simulink model "Acceleration_ANTTAY001"  (R2020a)
settings: Solver=ode4  StartTime=0.0  StopTime=45  FixedStep=0.2  RelTol=1e-3
model workspace (MAT data in the model file):
  alpha_gain = Simulink.Parameter
  alpha_gain.DataType = 'auto'
  alpha_gain.Dimensions = [0 0]
undefined symbols (not defined in the file or in its folder): K
settings Model: Creator=KNMALE002  LastModifiedBy=Tayla
settings DataIOCC: SaveOutput=off  SignalLogging=off  DSMLogging=off  ReturnWorkspaceOutputs=off  TimeSaveName=simulation_time
settings DebuggingCC: ArithmeticOperatorsInVariantConditions=warning
settings SFSimCC: CustomCodeUndefinedFunction=UseInterfaceOnly

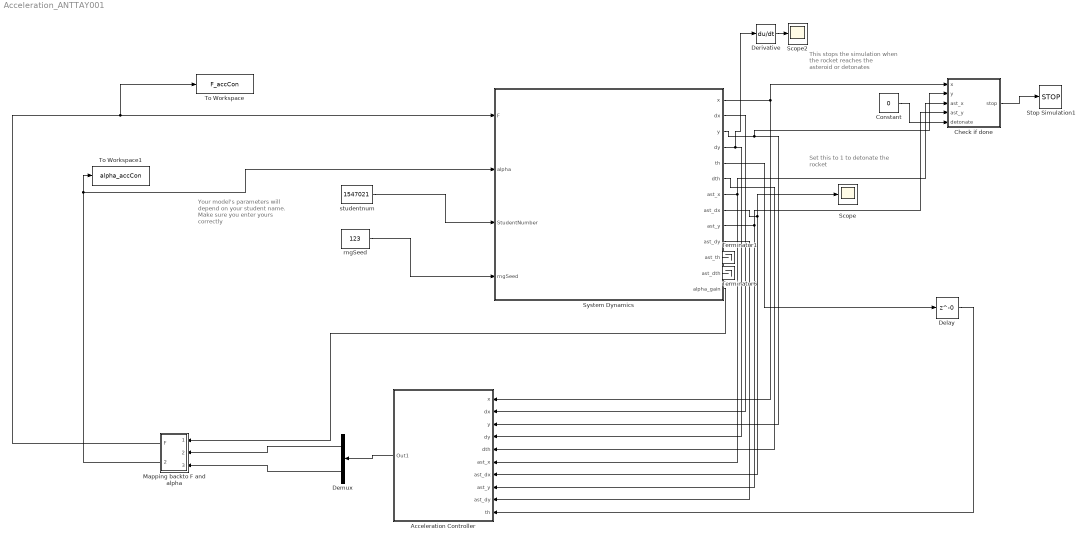
== system Acceleration_ANTTAY001 ==
  note: Your model's parameters will depend on your student name. Make sure you enter yours correctly
  note: This stops the simulation when the rocket reaches the asteroid or detonates
  note: Set this to 1 to detonate the rocket
  Acceleration Controller : Subsystem
  Check if done : MATLAB Function  TreatAsAtomicUnit=on
  Constant : Constant  Value=0
  Delay : Delay  DelayLength=0  InitialCondition=-pi/8
  Demux : Demux  Outputs=2
  Derivative : Derivative
  Mapping backto F and alpha : Subsystem
  Scope : Scope
  Scope2 : Scope
  Stop Simulation1 : Stop
  System Dynamics : Subsystem  TreatAsAtomicUnit=on  mask{Value=1}
      mask prompts: Value "Enter mode (1, 2 or 3)"
      mask TypeOptions Value: ScenarioVar/Value
      mask Display: image('lander.jpg');
  Terminator1 : Terminator
  Terminator6 : Terminator
  To Workspace : ToWorkspace  VariableName=F_accCon  SaveFormat=Timeseries  SampleTime=-1
  To Workspace1 : ToWorkspace  VariableName=alpha_accCon  SaveFormat=Timeseries  SampleTime=-1
  rngSeed : Constant  Value=123
  studentnum : Constant  Value=1547021
  wires:
  studentnum/1 -> System Dynamics/3(StudentNumber)
  System Dynamics/1(x) -> Check if done/1(x), Acceleration Controller/1(x)
  rngSeed/1 -> System Dynamics/4(rngSeed)
  System Dynamics/3(y) -> Acceleration Controller/3(y), Check if done/2(y)
  System Dynamics/9(ast_y) -> Check if done/4(ast_y), Acceleration Controller/8(ast_y)
  System Dynamics/8(ast_dx) -> Acceleration Controller/7(ast_dx), Scope/1
  Check if done/1(stop) -> Stop Simulation1/1
  Constant/1 -> Check if done/5(detonate)
  System Dynamics/4(dy) -> Derivative/1, Acceleration Controller/4(dy)
  Derivative/1 -> Scope2/1
  System Dynamics/7(ast_x) -> Acceleration Controller/6(ast_x), Check if done/3(ast_x)
  System Dynamics/11(ast_th) -> Terminator1/1
  System Dynamics/5(th) -> Delay/1
  System Dynamics/12(ast_dth) -> Terminator6/1
  System Dynamics/2(dx) -> Acceleration Controller/2(dx)
  System Dynamics/6(dth) -> Acceleration Controller/5(dth)
  System Dynamics/10(ast_dy) -> Acceleration Controller/9(ast_dy)
  Delay/1 -> Acceleration Controller/10(th)
  Acceleration Controller/1(Out1) -> Demux/1
  Mapping backto F and alpha/2(alpha) -> To Workspace1/1, System Dynamics/2(alpha)
  System Dynamics/13(alpha_gain) -> Mapping backto F and alpha/1(In1)
  Demux/1 -> Mapping backto F and alpha/2(In2)
  Demux/2 -> Mapping backto F and alpha/3(In3)
  Mapping backto F and alpha/1(F) -> System Dynamics/1(F), To Workspace/1

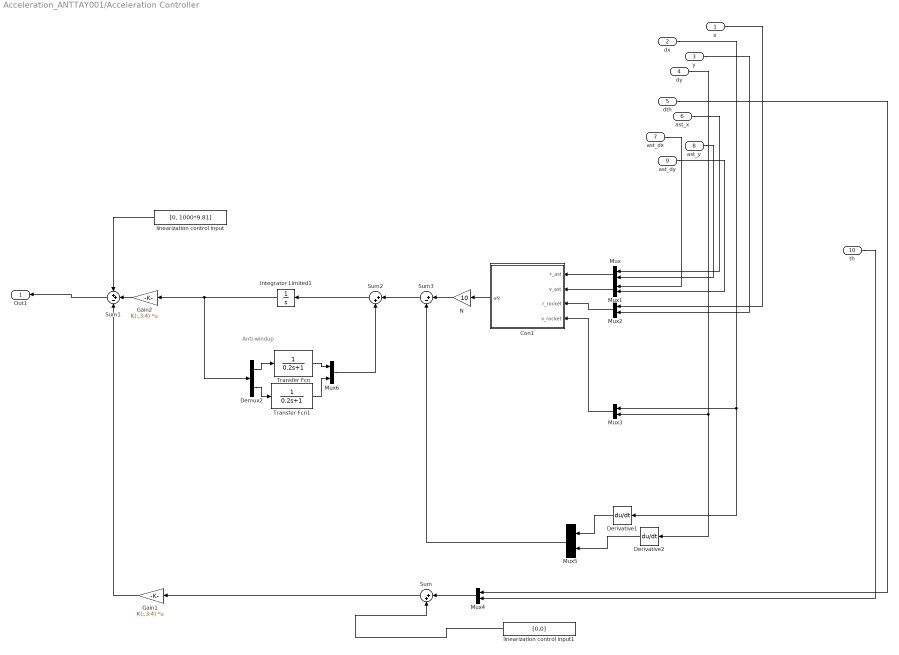
== system Acceleration_ANTTAY001/Acceleration Controller ==
  note: Anti-windup
  x : Inport
  dx : Inport  Port=2
  y : Inport  Port=3
  dy : Inport  Port=4
  dth : Inport  Port=5
  ast_x : Inport  Port=6
  ast_dx : Inport  Port=7
  ast_y : Inport  Port=8
  ast_dy : Inport  Port=9
  th : Inport  Port=10
  Con1 : MATLAB Function  TreatAsAtomicUnit=on
  Demux2 : Demux  Outputs=2
  Derivative1 : Derivative
  Derivative2 : Derivative
  Gain1 : Gain  Gain=K(:,3:4)  Multiplication=Matrix(K*u)
  Gain2 : Gain  Gain=K(:,3:4)  Multiplication=Matrix(K*u)
  Integrator Limited1 : Integrator  LimitOutput=on  UpperSaturationLimit=[8, 965]  LowerSaturationLimit=0
  Mux{,1..6} (7 alike) : Mux  Inputs=2
  N : Gain  Gain=10
  Sum : Sum  Inputs=|++
  Sum1 : Sum  Inputs=++-
  Sum2 : Sum  Inputs=|++
  Sum3 : Sum  Inputs=|+-
  Transfer Fcn : TransferFcn  Denominator=[0.2 1]
  Transfer Fcn1 : TransferFcn  Denominator=[0.2 1]
  linearization control input : Constant  Value=[0, 1000*9.81]
  linearization control input1 : Constant  Value=[0,0]
  Out1 : Outport
  wires:
  Mux5/1 -> Sum3/2
  Mux3/1 -> Con1/4(v_rocket)
  N/1 -> Sum3/1
  Mux/1 -> Con1/1(r_ast)
  Gain1/1 -> Sum1/3
  Mux1/1 -> Con1/2(v_ast)
  dy/1 -> Derivative2/1, Mux3/2
  Mux2/1 -> Con1/3(r_rocket)
  dx/1 -> Derivative1/1, Mux3/1
  dth/1 -> Mux4/1
  Gain2/1 -> Sum1/2
  ast_dx/1 -> Mux1/1
  Mux4/1 -> Sum/1
  Con1/1(aN) -> N/1
  y/1 -> Mux2/2
  Sum3/1 -> Sum2/1
  Derivative2/1 -> Mux5/2
  Derivative1/1 -> Mux5/1
  ast_dy/1 -> Mux1/2
  Sum2/1 -> Integrator Limited1/1
  linearization control input/1 -> Sum1/1
  x/1 -> Mux2/1
  linearization control input1/1 -> Sum/2
  Sum/1 -> Gain1/1
  ast_y/1 -> Mux/2
  ast_x/1 -> Mux/1
  Sum1/1 -> Out1/1
  th/1 -> Mux4/2
  Mux6/1 -> Sum2/2
  Transfer Fcn/1 -> Mux6/1
  Demux2/2 -> Transfer Fcn1/1
  Demux2/1 -> Transfer Fcn/1
  Integrator Limited1/1 -> Demux2/1, Gain2/1
  Transfer Fcn1/1 -> Mux6/2

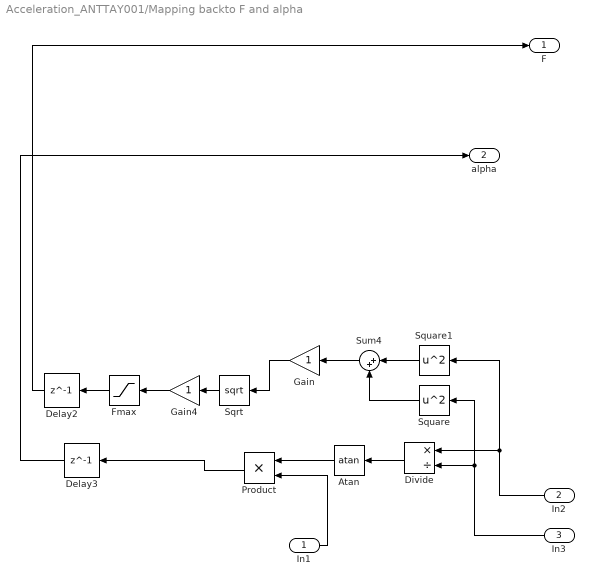
== system Acceleration_ANTTAY001/Mapping backto F and alpha ==
  In1 : Inport
  In2 : Inport  Port=2
  In3 : Inport  Port=3
  Atan : Trigonometry  Operator=atan
  Delay2 : Delay  DelayLength=1  InitialCondition=10000000000
  Delay3 : Delay  DelayLength=1
  Divide : Product  Inputs=*/
  Fmax : Saturate  UpperLimit=39250  LowerLimit=0
  Gain : Gain
  Gain4 : Gain
  Product : Product
  Sqrt : Sqrt  SaturateOnIntegerOverflow=on
  Square : Math  Operator=square  SignedPower=on  SaturateOnIntegerOverflow=on
  Square1 : Math  Operator=square  SignedPower=on  SaturateOnIntegerOverflow=on
  Sum4 : Sum  Inputs=|++
  F : Outport
  alpha : Outport  Port=2
  wires:
  Fmax/1 -> Delay2/1
  Sqrt/1 -> Gain4/1
  Divide/1 -> Atan/1
  In2/1 -> Divide/1, Square1/1
  Square1/1 -> Sum4/1
  Atan/1 -> Product/1
  Gain/1 -> Sqrt/1
  Sum4/1 -> Gain/1
  In3/1 -> Divide/2, Square/1
  Square/1 -> Sum4/2
  Gain4/1 -> Fmax/1
  Delay2/1 -> F/1
  Delay3/1 -> alpha/1
  Product/1 -> Delay3/1
  In1/1 -> Product/2

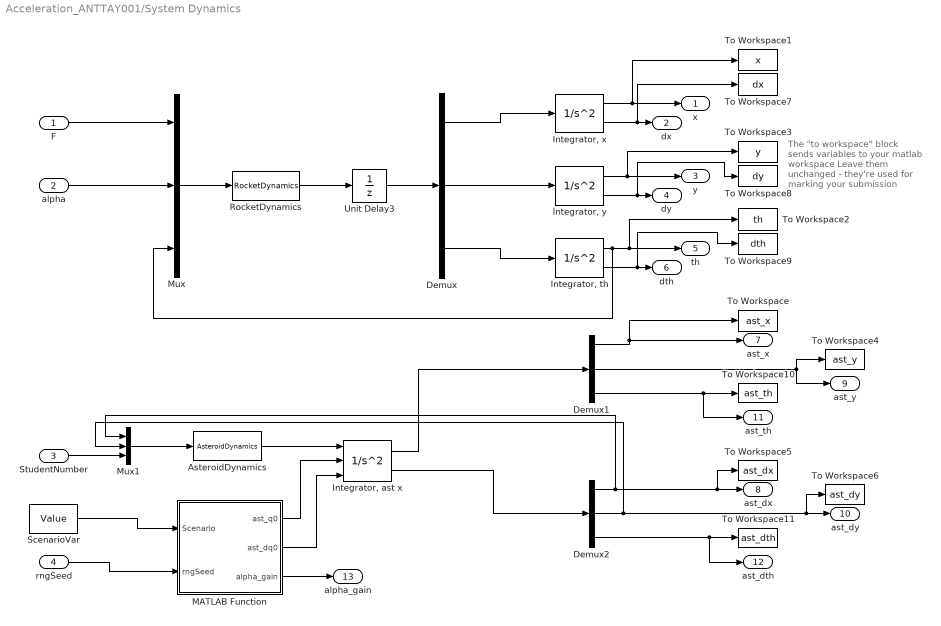
== system Acceleration_ANTTAY001/System Dynamics ==
  note: The "to workspace" block sends variables to your matlab workspace
      |
      | Leave them unchanged - they're used for marking your submission
  F : Inport
  alpha : Inport  Port=2
  StudentNumber : Inport  Port=3
  rngSeed : Inport  Port=4
  AsteroidDynamics : MATLABFcn  MATLABFcn=AsteroidDynamics  OutputDimensions=3
  Demux : Demux  Outputs=3
  Demux1 : Demux  Outputs=3
  Demux2 : Demux  Outputs=3
  "Integrator, th" : SecondOrderIntegrator  ICX=0  ICDXDT=0
  "Integrator, x" : SecondOrderIntegrator  ICX=0
  "Integrator, y" : SecondOrderIntegrator  ICX=0
  "Integrator, ast x" : SecondOrderIntegrator  ICSourceX=external  ICX=x0  ICSourceDXDT=external
  MATLAB Function : MATLAB Function  TreatAsAtomicUnit=on
  Mux : Mux  Inputs=3
  Mux1 : Mux  Inputs=3
  RocketDynamics : MATLABFcn  MATLABFcn=RocketDynamics  Output1D=off
  ScenarioVar : Constant  Value=Value
  To Workspace : ToWorkspace  VariableName=ast_x  SampleTime=-1
  To Workspace1 : ToWorkspace  VariableName=x  SampleTime=-1
  To Workspace10 : ToWorkspace  VariableName=ast_th  SampleTime=-1
  To Workspace11 : ToWorkspace  VariableName=ast_dth  SampleTime=-1
  To Workspace2 : ToWorkspace  VariableName=th  SampleTime=-1
  To Workspace3 : ToWorkspace  VariableName=y  SampleTime=-1
  To Workspace4 : ToWorkspace  VariableName=ast_y  SampleTime=-1
  To Workspace5 : ToWorkspace  VariableName=ast_dx  SampleTime=-1
  To Workspace6 : ToWorkspace  VariableName=ast_dy  SampleTime=-1
  To Workspace7 : ToWorkspace  VariableName=dx  SampleTime=-1
  To Workspace8 : ToWorkspace  VariableName=dy  SampleTime=-1
  To Workspace9 : ToWorkspace  VariableName=dth  SampleTime=-1
  Unit Delay3 : UnitDelay  SampleTime=-1  HasFrameUpgradeWarning=on
  x : Outport  PortDimensions=1  VectorParamsAs1DForOutWhenUnconnected=off
  dx : Outport  Port=2  PortDimensions=1  VectorParamsAs1DForOutWhenUnconnected=off
  y : Outport  Port=3  PortDimensions=1  VectorParamsAs1DForOutWhenUnconnected=off
  dy : Outport  Port=4  PortDimensions=1  VectorParamsAs1DForOutWhenUnconnected=off
  th : Outport  Port=5  PortDimensions=1  VectorParamsAs1DForOutWhenUnconnected=off
  dth : Outport  Port=6  PortDimensions=1  VectorParamsAs1DForOutWhenUnconnected=off
  ast_x : Outport  Port=7  PortDimensions=1  VectorParamsAs1DForOutWhenUnconnected=off
  ast_dx : Outport  Port=8  PortDimensions=1  VectorParamsAs1DForOutWhenUnconnected=off
  ast_y : Outport  Port=9  PortDimensions=1  VectorParamsAs1DForOutWhenUnconnected=off
  ast_dy : Outport  Port=10  PortDimensions=1  VectorParamsAs1DForOutWhenUnconnected=off
  ast_th : Outport  Port=11  PortDimensions=1  VectorParamsAs1DForOutWhenUnconnected=off
  ast_dth : Outport  Port=12  PortDimensions=1  VectorParamsAs1DForOutWhenUnconnected=off
  alpha_gain : Outport  Port=13
  wires:
  "Integrator, th"/1 -> th/1, To Workspace2/1, Mux/3
  Demux/1 -> "Integrator, x"/1
  Demux/2 -> "Integrator, y"/1
  Demux/3 -> "Integrator, th"/1
  "Integrator, x"/1 -> x/1, To Workspace1/1
  "Integrator, x"/2 -> To Workspace7/1, dx/1
  "Integrator, y"/2 -> To Workspace8/1, dy/1
  "Integrator, th"/2 -> To Workspace9/1, dth/1
  Mux/1 -> RocketDynamics/1
  RocketDynamics/1 -> Unit Delay3/1
  rngSeed/1 -> MATLAB Function/2(rngSeed)
  ScenarioVar/1 -> MATLAB Function/1(Scenario)
  F/1 -> Mux/1
  alpha/1 -> Mux/2
  Demux1/2 -> To Workspace4/1, ast_y/1
  Demux1/3 -> To Workspace10/1, ast_th/1
  Demux2/3 -> ast_dth/1, To Workspace11/1
  Mux1/1 -> AsteroidDynamics/1
  AsteroidDynamics/1 -> "Integrator, ast x"/1
  "Integrator, ast x"/1 -> Demux1/1
  "Integrator, ast x"/2 -> Demux2/1
  Demux1/1 -> To Workspace/1, ast_x/1
  Demux2/1 -> Mux1/1, To Workspace5/1, ast_dx/1
  Demux2/2 -> Mux1/2, To Workspace6/1, ast_dy/1
  MATLAB Function/1(ast_q0) -> "Integrator, ast x"/2
  MATLAB Function/2(ast_dq0) -> "Integrator, ast x"/3
  StudentNumber/1 -> Mux1/3
  Unit Delay3/1 -> Demux/1
  "Integrator, y"/1 -> y/1, To Workspace3/1
  MATLAB Function/3(alpha_gain) -> alpha_gain/1

== matlab function Acceleration_ANTTAY001/System Dynamics/MATLAB Function ==
  data: ast_q0 output; ast_dq0 output; Scenario input; rngSeed input; alpha_gain output
function [ast_q0, ast_dq0,alpha_gain] = fcn(Scenario, rngSeed)
rng(rngSeed);
alpha_gain = 1;

if (Scenario == 1)
    x0 = -3000;
    y0 =  5000;
    th0 =   0;
    dx0 = 182;
    dy0 = 0;
    dth0 = 0;
    alpha_gain = 1/10;
    
elseif (Scenario == 2)
    x0 = -2000 + rand_within_plus_minus(100);
    y0 = 4000 + rand_within_plus_minus(100); 
    th0 = 0;
    dx0 = 170;
    dy0 = 0;
    dth0 = 0.1;
    alpha_gain = 1;

elseif (Scenario == 3)
    x0 = -2500;
    y0 = 3000;
    th0 = 0;
    dx0 = 160;
    dy0 = 100;
    dth0 = deg2rad(rand_within_plus_minus(20)); % rad/sec
    theta_in = -pi/8;
    alpha_gain =1;
else
    error('You entered an invalid mode -- make sure Scenario = 1, 2 or 3')
end

alpha_gain = alpha_gain;
ast_q0  = [ x0;  y0;  th0];
ast_dq0 = [dx0; dy0; dth0];

end

% calling rand_within_plus_minus(100) returns a number between -100 and 100
function n = rand_within_plus_minus(interval)
    n = (rand - 0.5) * 2 * interval;
end

== matlab function Acceleration_ANTTAY001/Acceleration Controller/Con1 ==
  data: r_ast input; aN output size=2; v_ast input; r_rocket input; v_rocket input
function aN = pNav(r_ast, v_ast, r_rocket, v_rocket)
% https://en.wikipedia.org/wiki/Proportional_navigation
% this produces an acceleration which the controller should track
R = r_ast - r_rocket;
Rtemp = [R; 0];
Vr = v_ast - v_rocket;
Vtemp = [Vr; 0];
omega = cross(Rtemp, Vtemp) / dot(Rtemp, Rtemp);
temp = cross(Vtemp, omega);
aN = temp(1:2);

== matlab function Acceleration_ANTTAY001/Check if done ==
  data: x input; stop output; y input; ast_x input; ast_y input; detonate input
function stop = fcn(x, y, ast_x, ast_y, detonate)
    % given the signal to detonate
    if detonate == 1
        stop = 1;

    % rocket has hit the asteroid
    elseif norm([x; y] - [ast_x; ast_y]) < 100
        stop = 1;
    
    % rocket has hit the ground OR asteroid is close to they city
    elseif y < 0 || ast_y < 200
        stop = 1;
    
    else
        stop = 0;
    end
end
